simulink model "followWaypointsTrapVelTraj"  (R2020b)
settings: Solver=VariableStepAuto  StartTime=0.0  StopTime=inf  FixedStep=0.01  RelTol=1e-3  EnableMultiTasking=on
PreLoadFcn:
  | load('turtleBotMazeMap.mat')
libraries: simulink x1, mobileRoboticsLib x1, robotalgslib x1, robotcorelib x1, robotmobilelib x1
settings Model: Creator=scastro  LastModifiedBy=josea
settings DataIOCC: LimitDataPoints=on  ReturnWorkspaceOutputs=off
settings OptimizationCC: LifeSpan=inf
settings DebuggingCC: AllowSymbolicDim=off  SFUnexpectedBacktrackingDiag=warning  SFNoUnconditionalDefaultTransitionDiag=warning  SFExecutionAtInitializationDiag=none  ArithmeticOperatorsInVariantConditions=warning
settings SFSimCC: SimUseLocalCustomCode=off  CustomCodeUndefinedFunction=UseInterfaceOnly
settings RTWCC: RTWUseLocalCustomCode=off
settings CodeAppCC: StateflowObjectComments=on
settings GRTTargetCC: TargetLangStandard=C89/C90 (ANSI)
settings ConfigComp: CovMetricSettings=dw  CovSaveCumulativeToWorkspaceVar=on  CovSaveSingleToWorkspaceVar=on  CovExternalEMLEnable=off  CovSFcnEnable=off
settings SimscapeCC: SimscapeNominalValues="[{\"value\":\"10\",\"unit\":\"V\"},{\"value\":\"1\",\"unit\":\"A\"},{\"value\":\"10\",\"unit\":\"N*m\"},{\"value\":\"10\",\"unit\":\"bar\"},{\"value\":\"100\",\"unit\":\"kJ/kg\"},{\"value\":\"1\",\"unit\":\"kW\"},{\"value\":\"300\",\"unit\":\"K\"},{\"value\":\"100\",\"unit\":\"cm^3/s\"},{\"value\":\"1\",\"unit\":\"kN\"},{\"value\":\"1\",\"unit\":\"g/cm^3\"},{\"value\":\"1\",\"unit\":\"l\"},{\"value\":\"1\",\"unit\":\"cm^2\"},{\"value\":\"60\",\"unit\":\"Hz\"}]"  SimscapeLogType=all  SimscapeLogDataHistory=10000
settings ConfigurationSet: Description=SimMechanics 2G
settings ExplorerConfigSet: InternalSimMechanicsExplorerSettings="<ExplorerConfiguration><canonicalview>default</canonicalview><AnimationSetting><BasePlaybackSpeed>1.0</BasePlaybackSpeed><PlaybackSpeedFactor>1.0</PlaybackSpeedFactor></AnimationSetting><TilePanel><TileInfo><Tiles Columns=\"1\" Count=\"1\" Rows=\"1\"><Column Weight=\"1\"/><Row Weight=\"1\"/><Tile Height=\"1\" Width=\"1\" X=\"0\" Y=\"0\"/></Tiles></TileInfo><SceneInfo><SceneViewer><BGColor><R>0.60000002384185791</R><G>0.60000002384185791</G><B>0.60000002384185791</B></BGColor><Camera><DoPerspective>off</DoPerspective><Position><X>-1.70656042355848525</X><Y>-0.974920623359631922</Y><Z>4.72930454537082046</Z></Position><Center><X>0.552860638431633689</X><Y>1.42025063411503494</Y><Z>1.4843509506914252</Z></Center><Up><X>0.664249622453917166</X><Y>0.300615402055903091</Y><Z>0.684399604848363485</Z></Up><ViewLimDist>1</ViewLimDist><YLim>2.77881717169207398</YLim><XLim>3.55928742670435394</XLim></Camera></SceneViewer></SceneInfo></TilePanel><MechEditorPanel><Cameras/><GfxPanelCameraMap/><VideoCreator><PlaybackSpeedRatio>1.0</PlaybackSpeedRatio><FrameRate>30</FrameRate><VideoFormat>Motion JPEG AVI</VideoFormat><FrameSize>auto</FrameSize></VideoCreator></MechEditorPanel></ExplorerConfiguration>"

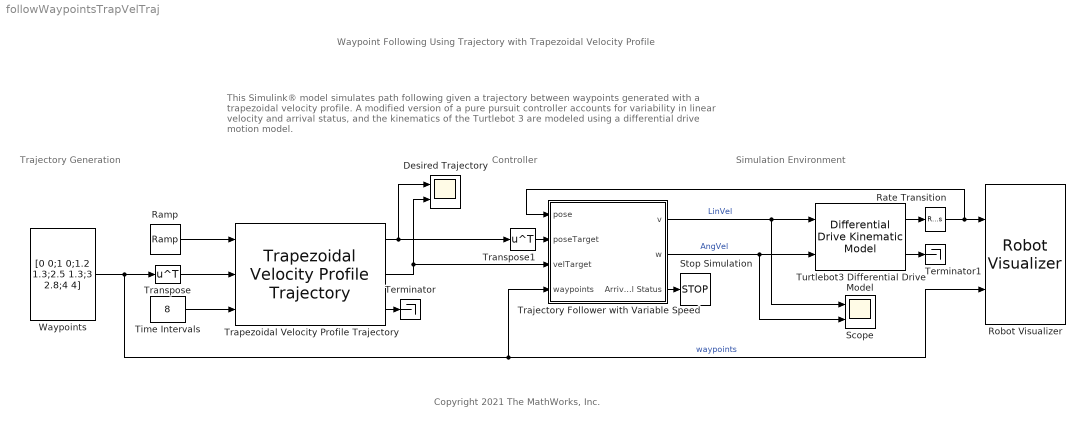
== system followWaypointsTrapVelTraj ==
  note: Simulation Environment
  note: Controller
  note: Trajectory Generation
  note: This Simulink® model simulates path following given a trajectory between waypoints generated with a trapezoidal velocity profile. A modified version of a pure pursuit controller accounts for variability in linear velocity and arrival status, and the kinematics of the Turtlebot 3 are modeled using a differential drive motion model.
  note: Copyright 2021 The MathWorks, Inc.
  note: Waypoint Following Using Trajectory with Trapezoidal Velocity Profile
  Desired Trajectory : Scope  NumInputPorts=2
  Ramp : simulink/Sources/Ramp  slope=1  start=0  InitialOutput=0
  Rate Transition : RateTransition  OutPortSampleTime=0.02
  Robot Visualizer : mobileRoboticsLib/Environments/Robot Visualizer  Priority=99  robotRadius=0.287  mapName=myOccMap  showTrajectory=on  hasWaypoints=on  hasLidar=off  sensorOffset=[0 0]  scanAngles=deg2rad(1:10:360)  hasObjDetector=off  objDetectorOffset=[ 0, 0 ]  objDetectorAngle=0  objDetectorFOV=0  objDetectorMaxRange=0  objectColors=0  objectMarkers='s'
  Scope : Scope  NumInputPorts=2
  Stop Simulation : Stop
  Terminator : Terminator
  Terminator1 : Terminator
  Time Intervals : Constant  Value=8
  Trajectory Follower with Variable Speed : Subsystem
  Transpose : Math  Operator=transpose  SaturateOnIntegerOverflow=on
  Transpose1 : Math  Operator=transpose  SaturateOnIntegerOverflow=on
  Trapezoidal Velocity Profile Trajectory : robotcorelib/Trapezoidal Velocity Profile Trajectory  WaypointSource=External  Waypoints=[ 0, -0.5, -1; 0, 0.5, 1 ]  NumParams=1  Parameter1=End Time  Parameter2=End Time  ParameterSource=External  PeakVelocity=[ 2; 2 ]  Acceleration=[ 1; 2 ]  EndTime=[ 1; 1 ]  AccelTime=[ 1; 2 ]  SimulateUsing=Code generation
      settings: SourceProductBaseCode=NV,RO,RR,UV
  Turtlebot3 Differential Drive Model : robotmobilelib/Differential Drive Kinematic Model  VehicleInputs=Vehicle Speed & Heading Angular Velocity  WheelRadius=0.033  WheelSpeedRange=[-inf inf]  TrackWidth=0.287  InitialState=[0; 0; 0]  SimulateUsing=Code generation
      settings: SourceProductBaseCode=RO
  Waypoints : Constant  Value=[0 0;1 0;1.2 1.3;2.5 1.3;3 2.8;4 4]
  wires:
  Waypoints/1 -> Trajectory Follower with Variable Speed/4(waypoints), Robot Visualizer/2, Transpose/1  "waypoints"
  Rate Transition/1 -> Trajectory Follower with Variable Speed/1(pose), Robot Visualizer/1
  Trajectory Follower with Variable Speed/1(v) -> Scope/1, Turtlebot3 Differential Drive Model/1  "LinVel"
  Trajectory Follower with Variable Speed/2(w) -> Turtlebot3 Differential Drive Model/2, Scope/2  "AngVel"
  Trajectory Follower with Variable Speed/3(Arrival Status) -> Stop Simulation/1
  Transpose/1 -> Trapezoidal Velocity Profile Trajectory/2
  Trapezoidal Velocity Profile Trajectory/1 -> Transpose1/1, Desired Trajectory/1
  Transpose1/1 -> Trajectory Follower with Variable Speed/2(poseTarget)
  Trapezoidal Velocity Profile Trajectory/2 -> Trajectory Follower with Variable Speed/3(velTarget), Desired Trajectory/2
  Ramp/1 -> Trapezoidal Velocity Profile Trajectory/1
  Time Intervals/1 -> Trapezoidal Velocity Profile Trajectory/3
  Trapezoidal Velocity Profile Trajectory/3 -> Terminator/1
  Turtlebot3 Differential Drive Model/1 -> Rate Transition/1
  Turtlebot3 Differential Drive Model/2 -> Terminator1/1

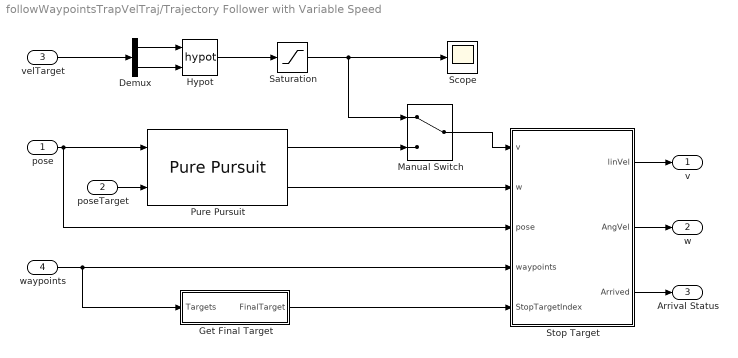
== system followWaypointsTrapVelTraj/Trajectory Follower with Variable Speed ==
  pose : Inport
  poseTarget : Inport  Port=2
  velTarget : Inport  Port=3
  waypoints : Inport  Port=4
  Demux : Demux  Outputs=2
  Get Final Target : Subsystem
  Hypot : Math  Operator=hypot  SaturateOnIntegerOverflow=on
  Manual Switch : ManualSwitch
  Pure Pursuit : robotalgslib/Pure Pursuit  DesiredLinearVelocity=0.26  MaxAngularVelocity=1.82  LookaheadDistance=0.05  TargetDirPort=off  SimulateUsing=Code generation
  Saturation : Saturate  UpperLimit=0.26  LowerLimit=0
  Scope : Scope
  Stop Target : Subsystem  mask(Stop at Target){threshold=0.22}
      mask prompts: threshold "Threshold Radius"
      mask help: This block takes in robot commands and a set of waypoints to set a velocity of zero when the robot pose compared to the waypoint is within the threshold specified.
  v : Outport  VectorParamsAs1DForOutWhenUnconnected=off
  w : Outport  Port=2  VectorParamsAs1DForOutWhenUnconnected=off
  Arrival Status : Outport  Port=3  VectorParamsAs1DForOutWhenUnconnected=off
  wires:
  pose/1 -> Pure Pursuit/1, Stop Target/3(pose)
  waypoints/1 -> Stop Target/4(waypoints), Get Final Target/1(Targets)
  Stop Target/3(Arrived) -> Arrival Status/1
  Get Final Target/1(FinalTarget) -> Stop Target/5(StopTargetIndex)
  Pure Pursuit/2 -> Stop Target/2(w)
  Pure Pursuit/1 -> Manual Switch/2
  Manual Switch/1 -> Stop Target/1(v)
  Stop Target/1(linVel) -> v/1
  Stop Target/2(AngVel) -> w/1
  poseTarget/1 -> Pure Pursuit/2
  velTarget/1 -> Demux/1
  Demux/1 -> Hypot/1
  Demux/2 -> Hypot/2
  Hypot/1 -> Saturation/1
  Saturation/1 -> Manual Switch/1, Scope/1

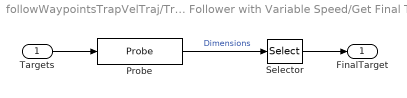
== system followWaypointsTrapVelTraj/Trajectory Follower with Variable Speed/Get Final Target ==
  Targets : Inport
  Probe : Probe  ProbeWidth=off  ProbeSampleTime=off  ProbeComplexSignal=off  ProbeSignalDimensions=on
  Selector : Selector  InputPortWidth=2  IndexOptions=Index vector (dialog)  Indices=1  OutputSizes=1
  FinalTarget : Outport
  wires:
  Probe/1 -> Selector/1  "Dimensions"
  Selector/1 -> FinalTarget/1
  Targets/1 -> Probe/1

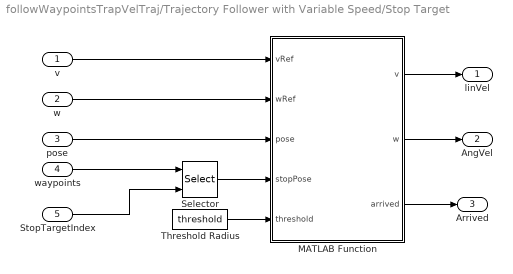
== system followWaypointsTrapVelTraj/Trajectory Follower with Variable Speed/Stop Target ==
  v : Inport
  w : Inport  Port=2
  pose : Inport  Port=3
  waypoints : Inport  Port=4
  StopTargetIndex : Inport  Port=5
  MATLAB Function : MATLAB Function  TreatAsAtomicUnit=on
  Selector : Selector  NumberOfDimensions=2  InputPortWidth=3  IndexOptions=Index vector (port),Index vector (dialog)  Indices=[1 3],[1 2]  OutputSizes=1,1
  Threshold Radius : Constant  Value=threshold
  linVel : Outport
  AngVel : Outport  Port=2
  Arrived : Outport  Port=3
  wires:
  v/1 -> MATLAB Function/1(vRef)
  Selector/1 -> MATLAB Function/4(stopPose)
  StopTargetIndex/1 -> Selector/2
  waypoints/1 -> Selector/1
  MATLAB Function/1(v) -> linVel/1
  pose/1 -> MATLAB Function/3(pose)
  w/1 -> MATLAB Function/2(wRef)
  Threshold Radius/1 -> MATLAB Function/5(threshold)
  MATLAB Function/3(arrived) -> Arrived/1
  MATLAB Function/2(w) -> AngVel/1

== matlab function followWaypointsTrapVelTraj/Trajectory Follower with Variable Speed/Stop Target/MATLAB Function ==
  data: v output; w output; vRef input; wRef input; pose input; stopPose input; threshold input; arrived output
function [v, w, arrived] = arrivalThreshold(vRef, wRef, pose, stopPose, threshold)

eucDist = sqrt((stopPose(1)-pose(1))^2 + (stopPose(2)-pose(2))^2);

if eucDist > threshold
    v = vRef;
    w = wRef;
    arrived = 0;
else
    v = 0;
    w = 0;
    arrived = 1;
end
